simulink model "PID_ThreeJoints"  (R2018b)
settings: Solver=FixedStepDiscrete  StartTime=0.0  StopTime=Inf  FixedStep=0.001  RelTol=1e-3  EnableMultiTasking=on
undefined symbols (not defined in the file): DiscIntNeverNeededParam, J1, J2, J3, J4, J5, J6, J7, Motor_Current, Motor_Position, Motor_Velocity, q, qd, Send_GUIdata, Tau
libraries: c280xlib x14, simulink x11, dspsrcs4 x6, idelinklib_common x1
(part 4 of 4)

== system PID_ThreeJoints/DynamicsController/DriveMotor/驱动器指令/Chart2/BG/J1_BG ==
  note: 命令
  note: 电流
  note: 位
      | 置
  Constant1 : Constant  Value=hex2dec('47')  OutDataTypeStr=uint8
  Constant2 : Constant  Value=0  VectorParams1D=off  OutDataTypeStr=uint8  SampleTime=-1
  Constant3 : Constant  Value=0  VectorParams1D=off  OutDataTypeStr=uint8  SampleTime=-1
  Constant8 : Constant  Value=hex2dec('42')  OutDataTypeStr=uint8
  Data Type Conversion : DataTypeConversion  OutDataTypeStr=uint16
  Data Type Conversion{1..6} (6 alike) : DataTypeConversion  OutDataTypeStr=uint8
  Mux3 : Mux  Inputs=8
  Shift Arithmetic1 : ArithShift  BitShiftNumber=8  BitShiftDirection=Right
  Shift Arithmetic2 : ArithShift  BitShiftNumber=16  BitShiftDirection=Right
  Shift Arithmetic3 : ArithShift  BitShiftNumber=24  BitShiftDirection=Right
  Shift Arithmetic4 : ArithShift  BitShiftNumber=8  BitShiftDirection=Right
  MSG : Outport
  wires:
  Shift Arithmetic2/1 -> Data Type Conversion4/1
  Shift Arithmetic4/1 -> Data Type Conversion6/1
  Constant2/1 -> Shift Arithmetic4/1, Data Type Conversion1/1
  Data Type Conversion1/1 -> Mux3/3
  Data Type Conversion3/1 -> Mux3/6
  Constant3/1 -> Data Type Conversion2/1, Shift Arithmetic1/1, Shift Arithmetic2/1, Shift Arithmetic3/1
  Data Type Conversion6/1 -> Mux3/4
  Shift Arithmetic3/1 -> Data Type Conversion5/1
  Shift Arithmetic1/1 -> Data Type Conversion3/1
  Mux3/1 -> Data Type Conversion/1
  Data Type Conversion2/1 -> Mux3/5
  Constant8/1 -> Mux3/1
  Data Type Conversion4/1 -> Mux3/7
  Data Type Conversion5/1 -> Mux3/8
  Constant1/1 -> Mux3/2
  Data Type Conversion/1 -> MSG/1

== system PID_ThreeJoints/DynamicsController/DriveMotor/驱动器指令/Chart2/BG/J2_BG ==
  note: 位
      | 置
  note: 电流
  note: 命令
  Constant1 : Constant  Value=hex2dec('47')  OutDataTypeStr=uint8
  Constant2 : Constant  Value=0  VectorParams1D=off  OutDataTypeStr=uint8  SampleTime=-1
  Constant3 : Constant  Value=0  VectorParams1D=off  OutDataTypeStr=uint8  SampleTime=-1
  Constant8 : Constant  Value=hex2dec('42')  OutDataTypeStr=uint8
  Data Type Conversion : DataTypeConversion  OutDataTypeStr=uint16
  Data Type Conversion{1..6} (6 alike) : DataTypeConversion  OutDataTypeStr=uint8
  Mux3 : Mux  Inputs=8
  Shift Arithmetic1 : ArithShift  BitShiftNumber=8  BitShiftDirection=Right
  Shift Arithmetic2 : ArithShift  BitShiftNumber=16  BitShiftDirection=Right
  Shift Arithmetic3 : ArithShift  BitShiftNumber=24  BitShiftDirection=Right
  Shift Arithmetic4 : ArithShift  BitShiftNumber=8  BitShiftDirection=Right
  MSG : Outport
  wires:
  Data Type Conversion/1 -> MSG/1
  Constant1/1 -> Mux3/2
  Data Type Conversion5/1 -> Mux3/8
  Data Type Conversion4/1 -> Mux3/7
  Constant8/1 -> Mux3/1
  Data Type Conversion2/1 -> Mux3/5
  Mux3/1 -> Data Type Conversion/1
  Shift Arithmetic1/1 -> Data Type Conversion3/1
  Shift Arithmetic3/1 -> Data Type Conversion5/1
  Data Type Conversion6/1 -> Mux3/4
  Constant3/1 -> Shift Arithmetic3/1, Shift Arithmetic2/1, Shift Arithmetic1/1, Data Type Conversion2/1
  Data Type Conversion3/1 -> Mux3/6
  Data Type Conversion1/1 -> Mux3/3
  Constant2/1 -> Data Type Conversion1/1, Shift Arithmetic4/1
  Shift Arithmetic4/1 -> Data Type Conversion6/1
  Shift Arithmetic2/1 -> Data Type Conversion4/1

== system PID_ThreeJoints/DynamicsController/DriveMotor/驱动器指令/Chart2/BG/J3_BG ==
  note: 命令
  note: 电流
  note: 位
      | 置
  Constant1 : Constant  Value=hex2dec('47')  OutDataTypeStr=uint8
  Constant2 : Constant  Value=0  VectorParams1D=off  OutDataTypeStr=uint8  SampleTime=-1
  Constant3 : Constant  Value=0  VectorParams1D=off  OutDataTypeStr=uint8  SampleTime=-1
  Constant8 : Constant  Value=hex2dec('42')  OutDataTypeStr=uint8
  Data Type Conversion : DataTypeConversion  OutDataTypeStr=uint16
  Data Type Conversion{1..6} (6 alike) : DataTypeConversion  OutDataTypeStr=uint8
  Mux3 : Mux  Inputs=8
  Shift Arithmetic1 : ArithShift  BitShiftNumber=8  BitShiftDirection=Right
  Shift Arithmetic2 : ArithShift  BitShiftNumber=16  BitShiftDirection=Right
  Shift Arithmetic3 : ArithShift  BitShiftNumber=24  BitShiftDirection=Right
  Shift Arithmetic4 : ArithShift  BitShiftNumber=8  BitShiftDirection=Right
  MSG : Outport
  wires:
  Shift Arithmetic2/1 -> Data Type Conversion4/1
  Shift Arithmetic4/1 -> Data Type Conversion6/1
  Constant2/1 -> Shift Arithmetic4/1, Data Type Conversion1/1
  Data Type Conversion1/1 -> Mux3/3
  Data Type Conversion3/1 -> Mux3/6
  Constant3/1 -> Data Type Conversion2/1, Shift Arithmetic1/1, Shift Arithmetic2/1, Shift Arithmetic3/1
  Data Type Conversion6/1 -> Mux3/4
  Shift Arithmetic3/1 -> Data Type Conversion5/1
  Shift Arithmetic1/1 -> Data Type Conversion3/1
  Mux3/1 -> Data Type Conversion/1
  Data Type Conversion2/1 -> Mux3/5
  Constant8/1 -> Mux3/1
  Data Type Conversion4/1 -> Mux3/7
  Data Type Conversion5/1 -> Mux3/8
  Constant1/1 -> Mux3/2
  Data Type Conversion/1 -> MSG/1

== system PID_ThreeJoints/DynamicsController/DriveMotor/驱动器指令/Chart2/BG/J4_BG ==
  note: 位
      | 置
  note: 电流
  note: 命令
  Constant1 : Constant  Value=hex2dec('47')  OutDataTypeStr=uint8
  Constant2 : Constant  Value=0  VectorParams1D=off  OutDataTypeStr=uint8  SampleTime=-1
  Constant3 : Constant  Value=0  VectorParams1D=off  OutDataTypeStr=uint8  SampleTime=-1
  Constant8 : Constant  Value=hex2dec('42')  OutDataTypeStr=uint8
  Data Type Conversion : DataTypeConversion  OutDataTypeStr=uint16
  Data Type Conversion{1..6} (6 alike) : DataTypeConversion  OutDataTypeStr=uint8
  Mux3 : Mux  Inputs=8
  Shift Arithmetic1 : ArithShift  BitShiftNumber=8  BitShiftDirection=Right
  Shift Arithmetic2 : ArithShift  BitShiftNumber=16  BitShiftDirection=Right
  Shift Arithmetic3 : ArithShift  BitShiftNumber=24  BitShiftDirection=Right
  Shift Arithmetic4 : ArithShift  BitShiftNumber=8  BitShiftDirection=Right
  MSG : Outport
  wires:
  Data Type Conversion/1 -> MSG/1
  Constant1/1 -> Mux3/2
  Data Type Conversion5/1 -> Mux3/8
  Data Type Conversion4/1 -> Mux3/7
  Constant8/1 -> Mux3/1
  Data Type Conversion2/1 -> Mux3/5
  Mux3/1 -> Data Type Conversion/1
  Shift Arithmetic1/1 -> Data Type Conversion3/1
  Shift Arithmetic3/1 -> Data Type Conversion5/1
  Data Type Conversion6/1 -> Mux3/4
  Constant3/1 -> Shift Arithmetic3/1, Shift Arithmetic2/1, Shift Arithmetic1/1, Data Type Conversion2/1
  Data Type Conversion3/1 -> Mux3/6
  Data Type Conversion1/1 -> Mux3/3
  Constant2/1 -> Data Type Conversion1/1, Shift Arithmetic4/1
  Shift Arithmetic4/1 -> Data Type Conversion6/1
  Shift Arithmetic2/1 -> Data Type Conversion4/1

== system PID_ThreeJoints/DynamicsController/DriveMotor/驱动器指令/Chart2/BG/J5_BG ==
  note: 命令
  note: 电流
  note: 位
      | 置
  Constant1 : Constant  Value=hex2dec('47')  OutDataTypeStr=uint8
  Constant2 : Constant  Value=0  VectorParams1D=off  OutDataTypeStr=uint8  SampleTime=-1
  Constant3 : Constant  Value=0  VectorParams1D=off  OutDataTypeStr=uint8  SampleTime=-1
  Constant8 : Constant  Value=hex2dec('42')  OutDataTypeStr=uint8
  Data Type Conversion : DataTypeConversion  OutDataTypeStr=uint16
  Data Type Conversion{1..6} (6 alike) : DataTypeConversion  OutDataTypeStr=uint8
  Mux3 : Mux  Inputs=8
  Shift Arithmetic1 : ArithShift  BitShiftNumber=8  BitShiftDirection=Right
  Shift Arithmetic2 : ArithShift  BitShiftNumber=16  BitShiftDirection=Right
  Shift Arithmetic3 : ArithShift  BitShiftNumber=24  BitShiftDirection=Right
  Shift Arithmetic4 : ArithShift  BitShiftNumber=8  BitShiftDirection=Right
  MSG : Outport
  wires:
  Shift Arithmetic2/1 -> Data Type Conversion4/1
  Shift Arithmetic4/1 -> Data Type Conversion6/1
  Constant2/1 -> Shift Arithmetic4/1, Data Type Conversion1/1
  Data Type Conversion1/1 -> Mux3/3
  Data Type Conversion3/1 -> Mux3/6
  Constant3/1 -> Data Type Conversion2/1, Shift Arithmetic1/1, Shift Arithmetic2/1, Shift Arithmetic3/1
  Data Type Conversion6/1 -> Mux3/4
  Shift Arithmetic3/1 -> Data Type Conversion5/1
  Shift Arithmetic1/1 -> Data Type Conversion3/1
  Mux3/1 -> Data Type Conversion/1
  Data Type Conversion2/1 -> Mux3/5
  Constant8/1 -> Mux3/1
  Data Type Conversion4/1 -> Mux3/7
  Data Type Conversion5/1 -> Mux3/8
  Constant1/1 -> Mux3/2
  Data Type Conversion/1 -> MSG/1

== system PID_ThreeJoints/DynamicsController/DriveMotor/驱动器指令/Chart2/BG/J6_BG ==
  note: 位
      | 置
  note: 电流
  note: 命令
  Constant1 : Constant  Value=hex2dec('47')  OutDataTypeStr=uint8
  Constant2 : Constant  Value=0  VectorParams1D=off  OutDataTypeStr=uint8  SampleTime=-1
  Constant3 : Constant  Value=0  VectorParams1D=off  OutDataTypeStr=uint8  SampleTime=-1
  Constant8 : Constant  Value=hex2dec('42')  OutDataTypeStr=uint8
  Data Type Conversion : DataTypeConversion  OutDataTypeStr=uint16
  Data Type Conversion{1..6} (6 alike) : DataTypeConversion  OutDataTypeStr=uint8
  Mux3 : Mux  Inputs=8
  Shift Arithmetic1 : ArithShift  BitShiftNumber=8  BitShiftDirection=Right
  Shift Arithmetic2 : ArithShift  BitShiftNumber=16  BitShiftDirection=Right
  Shift Arithmetic3 : ArithShift  BitShiftNumber=24  BitShiftDirection=Right
  Shift Arithmetic4 : ArithShift  BitShiftNumber=8  BitShiftDirection=Right
  MSG : Outport
  wires:
  Data Type Conversion/1 -> MSG/1
  Constant1/1 -> Mux3/2
  Data Type Conversion5/1 -> Mux3/8
  Data Type Conversion4/1 -> Mux3/7
  Constant8/1 -> Mux3/1
  Data Type Conversion2/1 -> Mux3/5
  Mux3/1 -> Data Type Conversion/1
  Shift Arithmetic1/1 -> Data Type Conversion3/1
  Shift Arithmetic3/1 -> Data Type Conversion5/1
  Data Type Conversion6/1 -> Mux3/4
  Constant3/1 -> Shift Arithmetic3/1, Shift Arithmetic2/1, Shift Arithmetic1/1, Data Type Conversion2/1
  Data Type Conversion3/1 -> Mux3/6
  Data Type Conversion1/1 -> Mux3/3
  Constant2/1 -> Data Type Conversion1/1, Shift Arithmetic4/1
  Shift Arithmetic4/1 -> Data Type Conversion6/1
  Shift Arithmetic2/1 -> Data Type Conversion4/1

== system PID_ThreeJoints/DynamicsController/DriveMotor/驱动器指令/Chart2/TF/J1_TF ==
  note: 命令
  note: 位
      | 置
  note: 电流
  Current : Inport
  Constant1 : Constant  Value=hex2dec('46')  OutDataTypeStr=uint8
  Constant3 : Constant  Value=0  VectorParams1D=off  OutDataTypeStr=uint8  SampleTime=-1
  Constant8 : Constant  Value=hex2dec('54')  OutDataTypeStr=uint8
  Data Type Conversion : DataTypeConversion  OutDataTypeStr=uint16
  Data Type Conversion{1..6} (6 alike) : DataTypeConversion  OutDataTypeStr=uint8
  Mux3 : Mux  Inputs=8
  Shift Arithmetic1 : ArithShift  BitShiftNumber=8  BitShiftDirection=Right
  Shift Arithmetic2 : ArithShift  BitShiftNumber=16  BitShiftDirection=Right
  Shift Arithmetic3 : ArithShift  BitShiftNumber=24  BitShiftDirection=Right
  Shift Arithmetic4 : ArithShift  BitShiftNumber=8  BitShiftDirection=Right
  MSG : Outport  OutDataTypeStr=uint16
  wires:
  Shift Arithmetic1/1 -> Data Type Conversion3/1
  Shift Arithmetic3/1 -> Data Type Conversion5/1
  Constant3/1 -> Shift Arithmetic3/1, Shift Arithmetic2/1, Shift Arithmetic1/1, Data Type Conversion2/1
  Mux3/1 -> Data Type Conversion/1
  Constant8/1 -> Mux3/1
  Data Type Conversion3/1 -> Mux3/6
  Data Type Conversion2/1 -> Mux3/5
  Data Type Conversion1/1 -> Mux3/3
  Data Type Conversion5/1 -> Mux3/8
  Current/1 -> Shift Arithmetic4/1, Data Type Conversion1/1
  Shift Arithmetic2/1 -> Data Type Conversion4/1
  Constant1/1 -> Mux3/2
  Data Type Conversion6/1 -> Mux3/4
  Shift Arithmetic4/1 -> Data Type Conversion6/1
  Data Type Conversion4/1 -> Mux3/7
  Data Type Conversion/1 -> MSG/1

== system PID_ThreeJoints/DynamicsController/DriveMotor/驱动器指令/Chart2/TF/J2_TF ==
  note: 电流
  note: 位
      | 置
  note: 命令
  Current : Inport
  Constant1 : Constant  Value=hex2dec('46')  OutDataTypeStr=uint8
  Constant3 : Constant  Value=0  VectorParams1D=off  OutDataTypeStr=uint8  SampleTime=-1
  Constant8 : Constant  Value=hex2dec('54')  OutDataTypeStr=uint8
  Data Type Conversion : DataTypeConversion  OutDataTypeStr=uint16
  Data Type Conversion{1..6} (6 alike) : DataTypeConversion  OutDataTypeStr=uint8
  Mux3 : Mux  Inputs=8
  Shift Arithmetic1 : ArithShift  BitShiftNumber=8  BitShiftDirection=Right
  Shift Arithmetic2 : ArithShift  BitShiftNumber=16  BitShiftDirection=Right
  Shift Arithmetic3 : ArithShift  BitShiftNumber=24  BitShiftDirection=Right
  Shift Arithmetic4 : ArithShift  BitShiftNumber=8  BitShiftDirection=Right
  MSG : Outport  OutDataTypeStr=uint16
  wires:
  Data Type Conversion/1 -> MSG/1
  Data Type Conversion4/1 -> Mux3/7
  Shift Arithmetic4/1 -> Data Type Conversion6/1
  Data Type Conversion6/1 -> Mux3/4
  Constant1/1 -> Mux3/2
  Shift Arithmetic2/1 -> Data Type Conversion4/1
  Current/1 -> Data Type Conversion1/1, Shift Arithmetic4/1
  Data Type Conversion5/1 -> Mux3/8
  Data Type Conversion1/1 -> Mux3/3
  Data Type Conversion2/1 -> Mux3/5
  Data Type Conversion3/1 -> Mux3/6
  Constant8/1 -> Mux3/1
  Mux3/1 -> Data Type Conversion/1
  Constant3/1 -> Data Type Conversion2/1, Shift Arithmetic1/1, Shift Arithmetic2/1, Shift Arithmetic3/1
  Shift Arithmetic3/1 -> Data Type Conversion5/1
  Shift Arithmetic1/1 -> Data Type Conversion3/1

== system PID_ThreeJoints/DynamicsController/DriveMotor/驱动器指令/Chart2/TF/J3_TF ==
  note: 命令
  note: 位
      | 置
  note: 电流
  Current : Inport
  Constant1 : Constant  Value=hex2dec('46')  OutDataTypeStr=uint8
  Constant3 : Constant  Value=0  VectorParams1D=off  OutDataTypeStr=uint8  SampleTime=-1
  Constant8 : Constant  Value=hex2dec('54')  OutDataTypeStr=uint8
  Data Type Conversion : DataTypeConversion  OutDataTypeStr=uint16
  Data Type Conversion{1..6} (6 alike) : DataTypeConversion  OutDataTypeStr=uint8
  Mux3 : Mux  Inputs=8
  Shift Arithmetic1 : ArithShift  BitShiftNumber=8  BitShiftDirection=Right
  Shift Arithmetic2 : ArithShift  BitShiftNumber=16  BitShiftDirection=Right
  Shift Arithmetic3 : ArithShift  BitShiftNumber=24  BitShiftDirection=Right
  Shift Arithmetic4 : ArithShift  BitShiftNumber=8  BitShiftDirection=Right
  MSG : Outport  OutDataTypeStr=uint16
  wires:
  Shift Arithmetic1/1 -> Data Type Conversion3/1
  Shift Arithmetic3/1 -> Data Type Conversion5/1
  Constant3/1 -> Shift Arithmetic3/1, Shift Arithmetic2/1, Shift Arithmetic1/1, Data Type Conversion2/1
  Mux3/1 -> Data Type Conversion/1
  Constant8/1 -> Mux3/1
  Data Type Conversion3/1 -> Mux3/6
  Data Type Conversion2/1 -> Mux3/5
  Data Type Conversion1/1 -> Mux3/3
  Data Type Conversion5/1 -> Mux3/8
  Current/1 -> Shift Arithmetic4/1, Data Type Conversion1/1
  Shift Arithmetic2/1 -> Data Type Conversion4/1
  Constant1/1 -> Mux3/2
  Data Type Conversion6/1 -> Mux3/4
  Shift Arithmetic4/1 -> Data Type Conversion6/1
  Data Type Conversion4/1 -> Mux3/7
  Data Type Conversion/1 -> MSG/1

== system PID_ThreeJoints/DynamicsController/DriveMotor/驱动器指令/Chart2/TF/J4_TF ==
  note: 电流
  note: 位
      | 置
  note: 命令
  Current : Inport
  Constant1 : Constant  Value=hex2dec('46')  OutDataTypeStr=uint8
  Constant3 : Constant  Value=0  VectorParams1D=off  OutDataTypeStr=uint8  SampleTime=-1
  Constant8 : Constant  Value=hex2dec('54')  OutDataTypeStr=uint8
  Data Type Conversion : DataTypeConversion  OutDataTypeStr=uint16
  Data Type Conversion{1..6} (6 alike) : DataTypeConversion  OutDataTypeStr=uint8
  Mux3 : Mux  Inputs=8
  Shift Arithmetic1 : ArithShift  BitShiftNumber=8  BitShiftDirection=Right
  Shift Arithmetic2 : ArithShift  BitShiftNumber=16  BitShiftDirection=Right
  Shift Arithmetic3 : ArithShift  BitShiftNumber=24  BitShiftDirection=Right
  Shift Arithmetic4 : ArithShift  BitShiftNumber=8  BitShiftDirection=Right
  MSG : Outport  OutDataTypeStr=uint16
  wires:
  Data Type Conversion/1 -> MSG/1
  Data Type Conversion4/1 -> Mux3/7
  Shift Arithmetic4/1 -> Data Type Conversion6/1
  Data Type Conversion6/1 -> Mux3/4
  Constant1/1 -> Mux3/2
  Shift Arithmetic2/1 -> Data Type Conversion4/1
  Current/1 -> Data Type Conversion1/1, Shift Arithmetic4/1
  Data Type Conversion5/1 -> Mux3/8
  Data Type Conversion1/1 -> Mux3/3
  Data Type Conversion2/1 -> Mux3/5
  Data Type Conversion3/1 -> Mux3/6
  Constant8/1 -> Mux3/1
  Mux3/1 -> Data Type Conversion/1
  Constant3/1 -> Data Type Conversion2/1, Shift Arithmetic1/1, Shift Arithmetic2/1, Shift Arithmetic3/1
  Shift Arithmetic3/1 -> Data Type Conversion5/1
  Shift Arithmetic1/1 -> Data Type Conversion3/1

== system PID_ThreeJoints/DynamicsController/DriveMotor/驱动器指令/Chart2/TF/J5_TF ==
  note: 命令
  note: 位
      | 置
  note: 电流
  Current : Inport
  Constant1 : Constant  Value=hex2dec('46')  OutDataTypeStr=uint8
  Constant3 : Constant  Value=0  VectorParams1D=off  OutDataTypeStr=uint8  SampleTime=-1
  Constant8 : Constant  Value=hex2dec('54')  OutDataTypeStr=uint8
  Data Type Conversion : DataTypeConversion  OutDataTypeStr=uint16
  Data Type Conversion{1..6} (6 alike) : DataTypeConversion  OutDataTypeStr=uint8
  Mux3 : Mux  Inputs=8
  Shift Arithmetic1 : ArithShift  BitShiftNumber=8  BitShiftDirection=Right
  Shift Arithmetic2 : ArithShift  BitShiftNumber=16  BitShiftDirection=Right
  Shift Arithmetic3 : ArithShift  BitShiftNumber=24  BitShiftDirection=Right
  Shift Arithmetic4 : ArithShift  BitShiftNumber=8  BitShiftDirection=Right
  MSG : Outport  OutDataTypeStr=uint16
  wires:
  Shift Arithmetic1/1 -> Data Type Conversion3/1
  Shift Arithmetic3/1 -> Data Type Conversion5/1
  Constant3/1 -> Shift Arithmetic3/1, Shift Arithmetic2/1, Shift Arithmetic1/1, Data Type Conversion2/1
  Mux3/1 -> Data Type Conversion/1
  Constant8/1 -> Mux3/1
  Data Type Conversion3/1 -> Mux3/6
  Data Type Conversion2/1 -> Mux3/5
  Data Type Conversion1/1 -> Mux3/3
  Data Type Conversion5/1 -> Mux3/8
  Current/1 -> Shift Arithmetic4/1, Data Type Conversion1/1
  Shift Arithmetic2/1 -> Data Type Conversion4/1
  Constant1/1 -> Mux3/2
  Data Type Conversion6/1 -> Mux3/4
  Shift Arithmetic4/1 -> Data Type Conversion6/1
  Data Type Conversion4/1 -> Mux3/7
  Data Type Conversion/1 -> MSG/1

== system PID_ThreeJoints/DynamicsController/DriveMotor/驱动器指令/Chart2/TF/J6_TF ==
  note: 电流
  note: 位
      | 置
  note: 命令
  Current : Inport
  Constant1 : Constant  Value=hex2dec('46')  OutDataTypeStr=uint8
  Constant3 : Constant  Value=0  VectorParams1D=off  OutDataTypeStr=uint8  SampleTime=-1
  Constant8 : Constant  Value=hex2dec('54')  OutDataTypeStr=uint8
  Data Type Conversion : DataTypeConversion  OutDataTypeStr=uint16
  Data Type Conversion{1..6} (6 alike) : DataTypeConversion  OutDataTypeStr=uint8
  Mux3 : Mux  Inputs=8
  Shift Arithmetic1 : ArithShift  BitShiftNumber=8  BitShiftDirection=Right
  Shift Arithmetic2 : ArithShift  BitShiftNumber=16  BitShiftDirection=Right
  Shift Arithmetic3 : ArithShift  BitShiftNumber=24  BitShiftDirection=Right
  Shift Arithmetic4 : ArithShift  BitShiftNumber=8  BitShiftDirection=Right
  MSG : Outport  OutDataTypeStr=uint16
  wires:
  Data Type Conversion/1 -> MSG/1
  Data Type Conversion4/1 -> Mux3/7
  Shift Arithmetic4/1 -> Data Type Conversion6/1
  Data Type Conversion6/1 -> Mux3/4
  Constant1/1 -> Mux3/2
  Shift Arithmetic2/1 -> Data Type Conversion4/1
  Current/1 -> Data Type Conversion1/1, Shift Arithmetic4/1
  Data Type Conversion5/1 -> Mux3/8
  Data Type Conversion1/1 -> Mux3/3
  Data Type Conversion2/1 -> Mux3/5
  Data Type Conversion3/1 -> Mux3/6
  Constant8/1 -> Mux3/1
  Mux3/1 -> Data Type Conversion/1
  Constant3/1 -> Data Type Conversion2/1, Shift Arithmetic1/1, Shift Arithmetic2/1, Shift Arithmetic3/1
  Shift Arithmetic3/1 -> Data Type Conversion5/1
  Shift Arithmetic1/1 -> Data Type Conversion3/1

== system PID_ThreeJoints/DynamicsController/DriveMotor/驱动器指令/Chart2/UM1/J1_UM1 ==
  note: 命令
  note: 位
      | 置
  note: 电流
  Constant1 : Constant  Value=hex2dec('4d')  OutDataTypeStr=uint8
  Constant2 : Constant  Value=0  VectorParams1D=off  OutDataTypeStr=uint8  SampleTime=-1
  Constant3 : Constant  VectorParams1D=off  OutDataTypeStr=uint8  SampleTime=-1
  Constant8 : Constant  Value=hex2dec('55')  OutDataTypeStr=uint8
  Data Type Conversion : DataTypeConversion  OutDataTypeStr=uint16
  Data Type Conversion{1..6} (6 alike) : DataTypeConversion  OutDataTypeStr=uint8
  Mux3 : Mux  Inputs=8
  Shift Arithmetic1 : ArithShift  BitShiftNumber=8  BitShiftDirection=Right
  Shift Arithmetic2 : ArithShift  BitShiftNumber=16  BitShiftDirection=Right
  Shift Arithmetic3 : ArithShift  BitShiftNumber=24  BitShiftDirection=Right
  Shift Arithmetic4 : ArithShift  BitShiftNumber=8  BitShiftDirection=Right
  MSG : Outport
  wires:
  Constant3/1 -> Shift Arithmetic3/1, Shift Arithmetic2/1, Data Type Conversion2/1, Shift Arithmetic1/1
  Data Type Conversion2/1 -> Mux3/5
  Data Type Conversion4/1 -> Mux3/7
  Mux3/1 -> Data Type Conversion/1
  Data Type Conversion6/1 -> Mux3/4
  Data Type Conversion/1 -> MSG/1
  Shift Arithmetic3/1 -> Data Type Conversion5/1
  Constant2/1 -> Data Type Conversion1/1, Shift Arithmetic4/1
  Data Type Conversion3/1 -> Mux3/6
  Constant8/1 -> Mux3/1
  Shift Arithmetic1/1 -> Data Type Conversion3/1
  Shift Arithmetic4/1 -> Data Type Conversion6/1
  Constant1/1 -> Mux3/2
  Data Type Conversion1/1 -> Mux3/3
  Shift Arithmetic2/1 -> Data Type Conversion4/1
  Data Type Conversion5/1 -> Mux3/8

== system PID_ThreeJoints/DynamicsController/DriveMotor/驱动器指令/Chart2/UM1/J2_UM1 ==
  note: 电流
  note: 位
      | 置
  note: 命令
  Constant1 : Constant  Value=hex2dec('4d')  OutDataTypeStr=uint8
  Constant2 : Constant  Value=0  VectorParams1D=off  OutDataTypeStr=uint8  SampleTime=-1
  Constant3 : Constant  VectorParams1D=off  OutDataTypeStr=uint8  SampleTime=-1
  Constant8 : Constant  Value=hex2dec('55')  OutDataTypeStr=uint8
  Data Type Conversion : DataTypeConversion  OutDataTypeStr=uint16
  Data Type Conversion{1..6} (6 alike) : DataTypeConversion  OutDataTypeStr=uint8
  Mux3 : Mux  Inputs=8
  Shift Arithmetic1 : ArithShift  BitShiftNumber=8  BitShiftDirection=Right
  Shift Arithmetic2 : ArithShift  BitShiftNumber=16  BitShiftDirection=Right
  Shift Arithmetic3 : ArithShift  BitShiftNumber=24  BitShiftDirection=Right
  Shift Arithmetic4 : ArithShift  BitShiftNumber=8  BitShiftDirection=Right
  MSG : Outport
  wires:
  Data Type Conversion5/1 -> Mux3/8
  Shift Arithmetic2/1 -> Data Type Conversion4/1
  Data Type Conversion1/1 -> Mux3/3
  Constant1/1 -> Mux3/2
  Shift Arithmetic4/1 -> Data Type Conversion6/1
  Shift Arithmetic1/1 -> Data Type Conversion3/1
  Constant8/1 -> Mux3/1
  Data Type Conversion3/1 -> Mux3/6
  Constant2/1 -> Shift Arithmetic4/1, Data Type Conversion1/1
  Shift Arithmetic3/1 -> Data Type Conversion5/1
  Data Type Conversion/1 -> MSG/1
  Data Type Conversion6/1 -> Mux3/4
  Mux3/1 -> Data Type Conversion/1
  Data Type Conversion4/1 -> Mux3/7
  Data Type Conversion2/1 -> Mux3/5
  Constant3/1 -> Shift Arithmetic1/1, Data Type Conversion2/1, Shift Arithmetic2/1, Shift Arithmetic3/1

== system PID_ThreeJoints/DynamicsController/DriveMotor/驱动器指令/Chart2/UM1/J3_UM1 ==
  note: 命令
  note: 位
      | 置
  note: 电流
  Constant1 : Constant  Value=hex2dec('4d')  OutDataTypeStr=uint8
  Constant2 : Constant  Value=0  VectorParams1D=off  OutDataTypeStr=uint8  SampleTime=-1
  Constant3 : Constant  VectorParams1D=off  OutDataTypeStr=uint8  SampleTime=-1
  Constant8 : Constant  Value=hex2dec('55')  OutDataTypeStr=uint8
  Data Type Conversion : DataTypeConversion  OutDataTypeStr=uint16
  Data Type Conversion{1..6} (6 alike) : DataTypeConversion  OutDataTypeStr=uint8
  Mux3 : Mux  Inputs=8
  Shift Arithmetic1 : ArithShift  BitShiftNumber=8  BitShiftDirection=Right
  Shift Arithmetic2 : ArithShift  BitShiftNumber=16  BitShiftDirection=Right
  Shift Arithmetic3 : ArithShift  BitShiftNumber=24  BitShiftDirection=Right
  Shift Arithmetic4 : ArithShift  BitShiftNumber=8  BitShiftDirection=Right
  MSG : Outport
  wires:
  Constant3/1 -> Shift Arithmetic3/1, Shift Arithmetic2/1, Data Type Conversion2/1, Shift Arithmetic1/1
  Data Type Conversion2/1 -> Mux3/5
  Data Type Conversion4/1 -> Mux3/7
  Mux3/1 -> Data Type Conversion/1
  Data Type Conversion6/1 -> Mux3/4
  Data Type Conversion/1 -> MSG/1
  Shift Arithmetic3/1 -> Data Type Conversion5/1
  Constant2/1 -> Data Type Conversion1/1, Shift Arithmetic4/1
  Data Type Conversion3/1 -> Mux3/6
  Constant8/1 -> Mux3/1
  Shift Arithmetic1/1 -> Data Type Conversion3/1
  Shift Arithmetic4/1 -> Data Type Conversion6/1
  Constant1/1 -> Mux3/2
  Data Type Conversion1/1 -> Mux3/3
  Shift Arithmetic2/1 -> Data Type Conversion4/1
  Data Type Conversion5/1 -> Mux3/8

== system PID_ThreeJoints/DynamicsController/DriveMotor/驱动器指令/Chart2/UM1/J4_UM1 ==
  note: 电流
  note: 位
      | 置
  note: 命令
  Constant1 : Constant  Value=hex2dec('4d')  OutDataTypeStr=uint8
  Constant2 : Constant  Value=0  VectorParams1D=off  OutDataTypeStr=uint8  SampleTime=-1
  Constant3 : Constant  VectorParams1D=off  OutDataTypeStr=uint8  SampleTime=-1
  Constant8 : Constant  Value=hex2dec('55')  OutDataTypeStr=uint8
  Data Type Conversion : DataTypeConversion  OutDataTypeStr=uint16
  Data Type Conversion{1..6} (6 alike) : DataTypeConversion  OutDataTypeStr=uint8
  Mux3 : Mux  Inputs=8
  Shift Arithmetic1 : ArithShift  BitShiftNumber=8  BitShiftDirection=Right
  Shift Arithmetic2 : ArithShift  BitShiftNumber=16  BitShiftDirection=Right
  Shift Arithmetic3 : ArithShift  BitShiftNumber=24  BitShiftDirection=Right
  Shift Arithmetic4 : ArithShift  BitShiftNumber=8  BitShiftDirection=Right
  MSG : Outport
  wires:
  Data Type Conversion5/1 -> Mux3/8
  Shift Arithmetic2/1 -> Data Type Conversion4/1
  Data Type Conversion1/1 -> Mux3/3
  Constant1/1 -> Mux3/2
  Shift Arithmetic4/1 -> Data Type Conversion6/1
  Shift Arithmetic1/1 -> Data Type Conversion3/1
  Constant8/1 -> Mux3/1
  Data Type Conversion3/1 -> Mux3/6
  Constant2/1 -> Shift Arithmetic4/1, Data Type Conversion1/1
  Shift Arithmetic3/1 -> Data Type Conversion5/1
  Data Type Conversion/1 -> MSG/1
  Data Type Conversion6/1 -> Mux3/4
  Mux3/1 -> Data Type Conversion/1
  Data Type Conversion4/1 -> Mux3/7
  Data Type Conversion2/1 -> Mux3/5
  Constant3/1 -> Shift Arithmetic1/1, Data Type Conversion2/1, Shift Arithmetic2/1, Shift Arithmetic3/1

== system PID_ThreeJoints/DynamicsController/DriveMotor/驱动器指令/Chart2/UM1/J5_UM1 ==
  note: 命令
  note: 位
      | 置
  note: 电流
  Constant1 : Constant  Value=hex2dec('4d')  OutDataTypeStr=uint8
  Constant2 : Constant  Value=0  VectorParams1D=off  OutDataTypeStr=uint8  SampleTime=-1
  Constant3 : Constant  VectorParams1D=off  OutDataTypeStr=uint8  SampleTime=-1
  Constant8 : Constant  Value=hex2dec('55')  OutDataTypeStr=uint8
  Data Type Conversion : DataTypeConversion  OutDataTypeStr=uint16
  Data Type Conversion{1..6} (6 alike) : DataTypeConversion  OutDataTypeStr=uint8
  Mux3 : Mux  Inputs=8
  Shift Arithmetic1 : ArithShift  BitShiftNumber=8  BitShiftDirection=Right
  Shift Arithmetic2 : ArithShift  BitShiftNumber=16  BitShiftDirection=Right
  Shift Arithmetic3 : ArithShift  BitShiftNumber=24  BitShiftDirection=Right
  Shift Arithmetic4 : ArithShift  BitShiftNumber=8  BitShiftDirection=Right
  MSG : Outport
  wires:
  Constant3/1 -> Shift Arithmetic3/1, Shift Arithmetic2/1, Data Type Conversion2/1, Shift Arithmetic1/1
  Data Type Conversion2/1 -> Mux3/5
  Data Type Conversion4/1 -> Mux3/7
  Mux3/1 -> Data Type Conversion/1
  Data Type Conversion6/1 -> Mux3/4
  Data Type Conversion/1 -> MSG/1
  Shift Arithmetic3/1 -> Data Type Conversion5/1
  Constant2/1 -> Data Type Conversion1/1, Shift Arithmetic4/1
  Data Type Conversion3/1 -> Mux3/6
  Constant8/1 -> Mux3/1
  Shift Arithmetic1/1 -> Data Type Conversion3/1
  Shift Arithmetic4/1 -> Data Type Conversion6/1
  Constant1/1 -> Mux3/2
  Data Type Conversion1/1 -> Mux3/3
  Shift Arithmetic2/1 -> Data Type Conversion4/1
  Data Type Conversion5/1 -> Mux3/8

== system PID_ThreeJoints/DynamicsController/DriveMotor/驱动器指令/Chart2/UM1/J6_UM1 ==
  note: 电流
  note: 位
      | 置
  note: 命令
  Constant1 : Constant  Value=hex2dec('4d')  OutDataTypeStr=uint8
  Constant2 : Constant  Value=0  VectorParams1D=off  OutDataTypeStr=uint8  SampleTime=-1
  Constant3 : Constant  VectorParams1D=off  OutDataTypeStr=uint8  SampleTime=-1
  Constant8 : Constant  Value=hex2dec('55')  OutDataTypeStr=uint8
  Data Type Conversion : DataTypeConversion  OutDataTypeStr=uint16
  Data Type Conversion{1..6} (6 alike) : DataTypeConversion  OutDataTypeStr=uint8
  Mux3 : Mux  Inputs=8
  Shift Arithmetic1 : ArithShift  BitShiftNumber=8  BitShiftDirection=Right
  Shift Arithmetic2 : ArithShift  BitShiftNumber=16  BitShiftDirection=Right
  Shift Arithmetic3 : ArithShift  BitShiftNumber=24  BitShiftDirection=Right
  Shift Arithmetic4 : ArithShift  BitShiftNumber=8  BitShiftDirection=Right
  MSG : Outport
  wires:
  Data Type Conversion5/1 -> Mux3/8
  Shift Arithmetic2/1 -> Data Type Conversion4/1
  Data Type Conversion1/1 -> Mux3/3
  Constant1/1 -> Mux3/2
  Shift Arithmetic4/1 -> Data Type Conversion6/1
  Shift Arithmetic1/1 -> Data Type Conversion3/1
  Constant8/1 -> Mux3/1
  Data Type Conversion3/1 -> Mux3/6
  Constant2/1 -> Shift Arithmetic4/1, Data Type Conversion1/1
  Shift Arithmetic3/1 -> Data Type Conversion5/1
  Data Type Conversion/1 -> MSG/1
  Data Type Conversion6/1 -> Mux3/4
  Mux3/1 -> Data Type Conversion/1
  Data Type Conversion4/1 -> Mux3/7
  Data Type Conversion2/1 -> Mux3/5
  Constant3/1 -> Shift Arithmetic1/1, Data Type Conversion2/1, Shift Arithmetic2/1, Shift Arithmetic3/1

== system PID_ThreeJoints/DynamicsController/DriveMotor/驱动器指令/Chart2/start_arm/StartRobotSubsystem ==
  In1 : Inport
  Enable : EnablePort
  System Outputs : Subsystem  mask(System Outputs){ShowInLibBrowser=0}
      mask prompts: ShowInLibBrowser "Simulink:masks:CustCodeMaskParam1_MP"
      settings: CopyFcn=cccopyfcn(gcb)  OpenFcn=ccopenfcn('System Outputs Function')
      mask Help: eval('feval(''rtwprivate'',''rtwhelpview'',''rtw_sys_outputs_block'')');
      mask DialogControl ShowInLibBrowser Prompt: Mask Parameter 1:
      mask Display: disp('System\nOutputs');
  Out1 : Outport
  wires:
  In1/1 -> Out1/1

== system PID_ThreeJoints/DynamicsController/DriveMotor/驱动器指令/Chart2/start_arm/StartRobotSubsystem/System Outputs ==

== stateflow chart PID_ThreeJoints/DynamicsController/DriveMotor/驱动器指令/Chart2 ==
  state bx = check(write) [function]
  state MSG = UM1 [function]
  state start = start_arm(StartRobot) [function]
  state State05
    entry:
    start=0;
    during:
    start=start_arm(StartRobot);
    %启动机械臂
  state State01
    entry:
    bx=0;
    during:
    bx=check(write);
  state State06
    entry:
    MSG = UM1;
  state State03
    entry:
    MSG = BG;
  state MSG = TF(Current) [function]
  state State04
    entry:
    during:
    MSG = TF(Current);
  state MSG = BG [function]
  State01 -> State06 : [bx>0]
  (default) -> State05
  State05 -> State01 : [start>0]
  State06 -> State03
  State03 -> State04
  data: write function_input uint16 size=1; bx function_output uint16 size=1; MSG function_output; StartRobot function_input uint16 size=1; start function_output uint16 size=1; MSG function_output; Current function_input uint16 size=[1 6]; MSG function_output; MSG output; Current input size=[1 6]; write input uint16 size=1; bx local uint16 size=1; start local uint16; StartRobot input uint16
